simulink model "ruf"  (R2024b)
settings: Solver=VariableStepAuto  StartTime=0.0  StopTime=50  RelTol=1e-3
libraries: spspowerguiLib x1
settings Model: Creator=Jatay  LastModifiedBy=Jatay

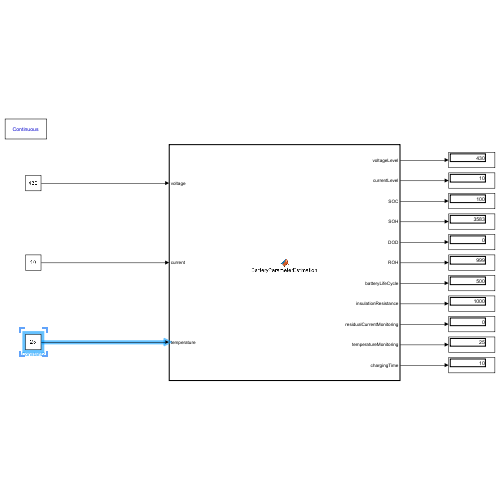
[thumbnail: Simulink's stored preview of the top-level diagram]
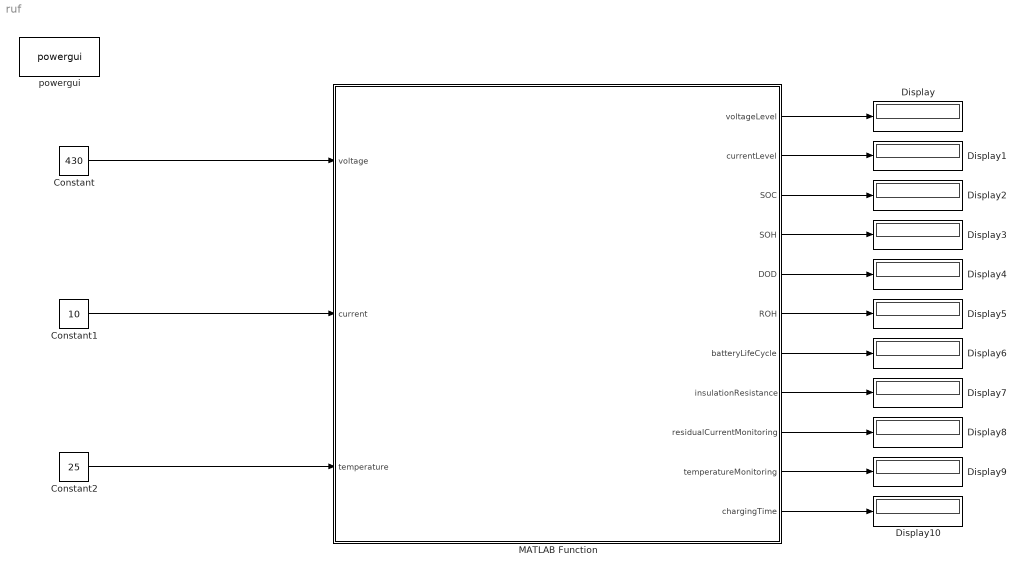
== system ruf ==
  Constant : Constant  Value=430
  Constant1 : Constant  Value=10
  Constant2 : Constant  Value=25
  Display{,1..10} (11 alike) : Display
  MATLAB Function : MATLAB Function  TreatAsAtomicUnit=on
  powergui : spspowerguiLib/powergui  Priority=1  SimulationMode=Continuous  SampleTime=50e-6  frequency=60  Iterations=50  frequencyindice=60  Pbase=100e6  ErrMax=1e-4  UnitsV=kV  UnitsW=MW  buscounter=0  FunctionMessages=off  echomessages=off  EnableUseOfTLC=off  CurrentSourceSwitches=off  DisableSnubberDevices=off  DisableRonSwitches=off  DisableVfSwitches=off  DisplayEquations=off  AutomaticDiscreteSolvers=off  SolverType=Tustin/Backward Euler (TBE)  Interpol=off  ExternalGateDelay=off  methode=off  Ts=100  x0status=blocks  SPID=on  SwTol=0  HookPort=off  NonlinearTolerance=1e-4  nMaxIteration=100  ContinueOnMaxIteration=off  RestoreLinks=warning  ResistiveCurrentMeasurement=off  Frange=[0:2:500]  Ylog=off  Xlog=on  ShowGrid=off  save=off  variable=ZData  structure=0  ZoomFFT=off  StartTime=0.0  cycles=1  DisplayStyle=1  fundamental=60  FreqAxis=off  MaxFrequency=1000  frequencyindicesteady=1  RmsSteady=1  display=off
  wires:
  Constant/1 -> MATLAB Function/1(voltage)
  Constant1/1 -> MATLAB Function/2(current)
  Constant2/1 -> MATLAB Function/3(temperature)
  MATLAB Function/1(voltageLevel) -> Display/1
  MATLAB Function/2(currentLevel) -> Display1/1
  MATLAB Function/3(SOC) -> Display2/1
  MATLAB Function/4(SOH) -> Display3/1
  MATLAB Function/5(DOD) -> Display4/1
  MATLAB Function/6(ROH) -> Display5/1
  MATLAB Function/7(batteryLifeCycle) -> Display6/1
  MATLAB Function/8(insulationResistance) -> Display7/1
  MATLAB Function/9(residualCurrentMonitoring) -> Display8/1
  MATLAB Function/10(temperatureMonitoring) -> Display9/1
  MATLAB Function/11(chargingTime) -> Display10/1

== matlab function ruf/MATLAB Function ==
  data: voltage input; voltageLevel output; current input; temperature input; currentLevel output; SOC output; SOH output; DOD output; ROH output; batteryLifeCycle output; insulationResistance output; residualCurrentMonitoring output; temperatureMonitoring output; chargingTime output
function [voltageLevel, currentLevel, SOC, SOH, DOD, ROH, batteryLifeCycle, insulationResistance, residualCurrentMonitoring, temperatureMonitoring, chargingTime] = BatteryParameterEstimation(voltage, current, temperature)
    % BatteryParameterEstimation calculates various battery parameters based on voltage, current, and temperature.
    %
    % Inputs:
    %   voltage - The voltage of the battery in volts
    %   current - The current flowing into the battery in amperes
    %   temperature - The temperature of the battery in degrees Celsius
    %
    % Outputs:
    %   voltageLevel - Monitored voltage level
    %   currentLevel - Monitored current level
    %   SOC - State of Charge as a percentage
    %   SOH - State of Health as a percentage
    %   DOD - Depth of Discharge as a percentage
    %   ROH - Remaining Operating Hours
    %   batteryLifeCycle - Estimated remaining battery life cycles
    %   insulationResistance - Insulation resistance in ohms (example constant)
    %   residualCurrentMonitoring - Boolean indicating overcurrent condition
    %   temperatureMonitoring - Monitored temperature value
    %   chargingTime - Estimated charging time in hours

    % Constants for calculations (these values are examples and may need to be adjusted)
    nominalVoltage = 12;        % Nominal voltage of the battery in volts
    maxCurrent = 100;           % Maximum current rating in amperes
    fullChargeCapacity = 100;   % Full charge capacity in Ah
    minVoltageCutoff = 10.5;    % Minimum voltage cutoff for the battery in volts
    maxCycles = 500;            % Estimated maximum cycles for the battery life

    %% 1. Voltage Levels
    voltageLevel = voltage;

    %% 2. Current Levels
    currentLevel = current;

    %% 3. State of Charge (SOC) Calculation
    SOC = (voltage - minVoltageCutoff) / (nominalVoltage - minVoltageCutoff) * 100;
    SOC = max(0, min(SOC, 100));  % Ensure SOC is between 0% and 100%

    %% 4. State of Health (SOH) Calculation (example based on voltage drop)
    SOH = (voltage / nominalVoltage) * 100;

    %% 5. Depth of Discharge (DOD) Calculation
    DOD = 100 - SOC;  % DOD is the complement of SOC

    %% 6. Remaining Operating Hours (ROH) Calculation
    ROH = (fullChargeCapacity - (current / fullChargeCapacity)) * fullChargeCapacity / current; 
    ROH = max(0, ROH);  % Ensure ROH is not negative

    %% 7. Battery Life Cycle Calculation
    batteryLifeCycle = maxCycles * (SOC / 100);  % Estimate remaining cycles based on SOC

    %% 8. Insulation Resistance Calculation (example constant)
    insulationResistance = 1000;  % Example value in ohms

    %% 9. Residual Current Monitoring Calculation (example condition)
    residualCurrentMonitoring = current > maxCurrent;  % True if overcurrent condition

    %% 10. Temperature Monitoring
    temperatureMonitoring = temperature;  % Directly use temperature input

    %% 11. Charging Time Calculation (example)
    chargingTime = (fullChargeCapacity - DOD * fullChargeCapacity / 100) / current; 
end
